simulink model "final_part4"  (R2023a)
settings: Solver=VariableStepAuto  StartTime=0.0  StopTime=10.0  RelTol=1e-3
values from neighbouring files (symbols this model uses):
  a = 81.44    [DetermineTorqConstants.m]    (also in part4.m = 69.9384142006)
  K = place (A,B, p)    [part4.m]
libraries: c6xlib x2, fricblocks x1
settings Model: Creator=rawnies2  LastModifiedBy=rawnies2

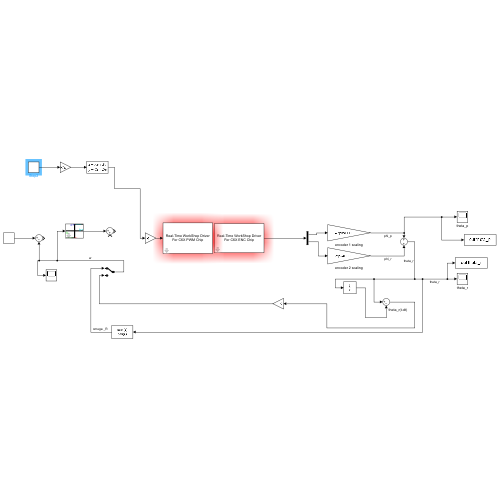
[thumbnail: Simulink's stored preview of the top-level diagram]
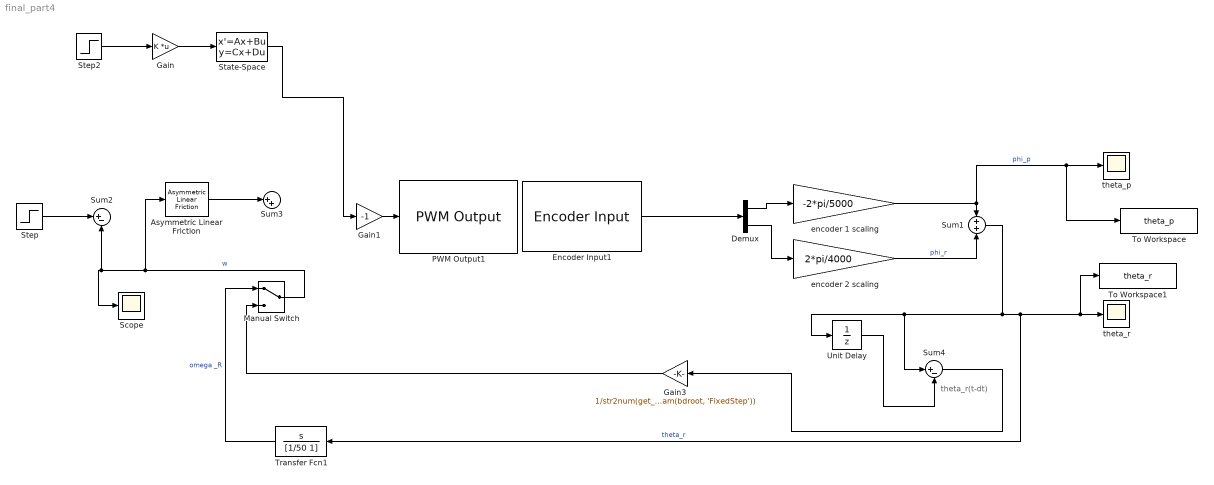
== system final_part4 ==
  note: theta_r(t-dt)
  Asymmetric Linear Friction : fricblocks/Asymmetric  Linear Friction  intercept1=0.6043  intercept2=-0.6143  slope1=0.01219  slope2=0.01291
  Demux : Demux  Outputs=2
  Encoder Input1 : c6xlib/Encoder Input  baseAddr=findParallelAddress  channels=[0 1]  sampleTime=str2num(get_param(bdroot, 'FixedStep'))
  Gain : Gain  Gain=K  Multiplication=Matrix(K*u)
  Gain1 : Gain  Gain=-1
  Gain3 : Gain  Gain=1/str2num(get_param(bdroot, 'FixedStep'))
  Manual Switch : ManualSwitch
  PWM Output1 : c6xlib/PWM Output  baseAddr=findParallelAddress  channels=0  initialOutputs=0  finalOutputs=0  sampleTime=str2num(get_param(bdroot, 'FixedStep'))
  Scope : Scope
  State-Space : StateSpace  A="[ 0 1  ; a 0 ];"  B=[ 0; -0.87];  C=[ 0 0;0 0]  D=[ 0 ;0]  InitialCondition=0
  Step : Step  Time=0  After=5  SampleTime=0
  Step2 : Step  Time=0  After=5  SampleTime=0
  Sum1 : Sum
  Sum2 : Sum  Inputs=|+-
  Sum3 : Sum  Inputs=|++
  Sum4 : Sum  Inputs=|+-
  To Workspace : ToWorkspace  VariableName=theta_p  SaveFormat=Structure With Time  SampleTime=-1
  To Workspace1 : ToWorkspace  VariableName=theta_r  SaveFormat=Structure With Time  SampleTime=-1
  Transfer Fcn1 : TransferFcn  Numerator=[1 0]  Denominator=[1/50 1]
  Unit Delay : UnitDelay  SampleTime=-1  HasFrameUpgradeWarning=on
  encoder 1 scaling : Gain  Gain=-2*pi/5000
  encoder 2 scaling : Gain  Gain=2*pi/4000
  theta_p : Scope
  theta_r : Scope
  wires:
  Unit Delay/1 -> Sum4/2
  Step/1 -> Sum2/1
  Gain1/1 -> PWM Output1/1
  Sum1/1 -> Sum4/1, Unit Delay/1, Transfer Fcn1/1, To Workspace1/1, theta_r/1  "theta_r"
  Demux/2 -> encoder 2 scaling/1
  Demux/1 -> encoder 1 scaling/1
  Manual Switch/1 -> Asymmetric Linear Friction/1, Scope/1, Sum2/2  "w"
  encoder 2 scaling/1 -> Sum1/2  "phi_r"
  Transfer Fcn1/1 -> Manual Switch/1  "omega _R"
  Gain3/1 -> Manual Switch/2
  Sum4/1 -> Gain3/1
  Encoder Input1/1 -> Demux/1
  Asymmetric Linear Friction/1 -> Sum3/1
  encoder 1 scaling/1 -> To Workspace/1, theta_p/1, Sum1/1  "phi_p"
  State-Space/1 -> Gain1/1
  Gain/1 -> State-Space/1
  Step2/1 -> Gain/1
